simulink model "lab7class"  (R2018a)
settings: Solver=VariableStepAuto  StartTime=0.0  StopTime=1  RelTol=1e-3
settings Model: Creator=symih  LastModifiedBy=symih

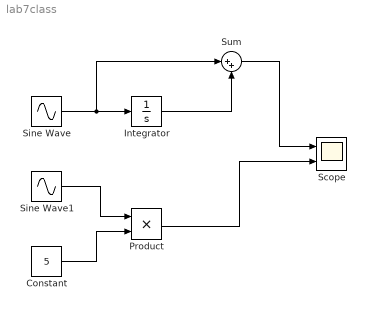
== system lab7class ==
  Constant : Constant  Value=5
  Integrator : Integrator
  Product : Product
  Scope : Scope  NumInputPorts=2
  Sine Wave : Sin  Amplitude=10  Frequency=2*pi*5  SampleTime=0.001
  Sine Wave1 : Sin  Amplitude=10  Frequency=2*pi*5  SampleTime=0.001
  Sum : Sum  Inputs=|++
  wires:
  Sine Wave/1 -> Sum/1, Integrator/1
  Integrator/1 -> Sum/2
  Sine Wave1/1 -> Product/1
  Constant/1 -> Product/2
  Product/1 -> Scope/2
  Sum/1 -> Scope/1
